simulink model "asgnmnt2_"  (Simulink 9.1)
settings: Solver=ode45  StartTime=0.0  StopTime=15.0  RelTol=1e-3  AbsTol=1e-3
settings Model: Creator=ewk15101  LastModifiedBy=ewk15101
settings DataIOCC: SaveFormat=Dataset
settings OptimizationCC: LifeSpan=auto
settings DebuggingCC: UnderspecifiedInitializationDetection=Simplified  MergeDetectMultiDrivingBlocksExec=error  SFUnexpectedBacktrackingDiag=error  SFNoUnconditionalDefaultTransitionDiag=error  SFExecutionAtInitializationDiag=warning
settings HardwareCC: ProdBitPerPointer=64  ProdBitPerSizeT=64  ProdBitPerPtrDiffT=64  ProdLargestAtomicFloat=Float  ProdIntDivRoundTo=Zero  ProdEndianess=LittleEndian  ProdWordSize=64  ProdHWDeviceType=Intel->x86-64 (Windows64)
settings ModelReferenceCC: PropagateSignalLabelsOutOfModel=on
settings CodeAppCC: StateflowObjectComments=off
settings GRTTargetCC: TargetLangStandard=C99 (ISO)  CombineOutputUpdateFcns=on  GRTInterface=off
settings ConfigComp: CovMetricSettings=dwe  CovHtmlReporting=off  CovSaveCumulativeToWorkspaceVar=off  CovSaveSingleToWorkspaceVar=off  CovExternalEMLEnable=on

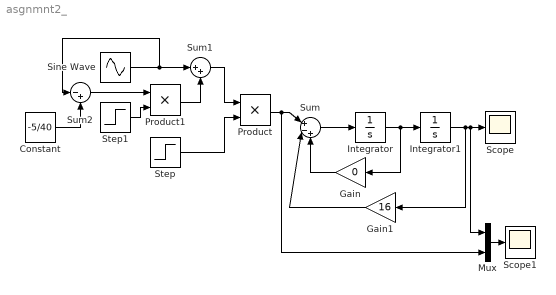
== system asgnmnt2_ ==
  Constant : Constant  Value=-5/40
  Gain : Gain  Gain=0
  Gain1 : Gain  Gain=16
  Integrator : Integrator
  Integrator1 : Integrator
  Mux : Mux  Inputs=2
  Product : Product
  Product1 : Product
  Scope : Scope
  Scope1 : Scope
  Sine Wave : Sin  Amplitude=5/40  Frequency=5  SampleTime=0
  Step : Step  Time=9  Before=1  After=0  SampleTime=0
  Step1 : Step  Time=1.5*pi  SampleTime=0
  Sum : Sum  Inputs=|+-+
  Sum1 : Sum  Inputs=|++
  Sum2 : Sum  Inputs=|-+
  wires:
  Integrator/1 -> Gain/1, Integrator1/1
  Sum/1 -> Integrator/1
  Sum1/1 -> Product/1
  Product/1 -> Mux/2, Sum/1
  Step/1 -> Product/2
  Sine Wave/1 -> Sum2/1, Sum1/1
  Integrator1/1 -> Mux/1, Scope/1, Gain1/1
  Gain1/1 -> Sum/2
  Gain/1 -> Sum/3
  Step1/1 -> Product1/2
  Product1/1 -> Sum1/2
  Constant/1 -> Sum2/2
  Sum2/1 -> Product1/1
  Mux/1 -> Scope1/1
